simulink model "SecRwRtStZeroTrgtPosSelc"  (R2018b)
settings: Solver=FixedStepDiscrete  StartTime=0.0  StopTime=10.0  RelTol=1e-3
undefined symbols (not defined in the file or in its folder): KeSMSw6SAcsEntrySecRwRtStCushnFrtUpwdDnwdPos_Val, KeSMSw6SAcsEntrySecRwRtStCushnFrtUpwdDnwdPosMax_Val, KeSMSw6SAcsEntrySecRwRtStCushnFrtUpwdDnwdPosMin_Val, KeSMSw6SRecoveryMdSecRwRtStCushnFrtUpwdDnwdPos_Val, KeSMSw6SRecoveryMdSecRwRtStCushnFrtUpwdDnwdPosMax_Val, KeSMSw6SRecoveryMdSecRwRtStCushnFrtUpwdDnwdPosMin_Val, KeSMSwAcsEntrySecRwRtStCushnFrtIUpwdDnwdPos_Val, KeSMSwAcsEntrySecRwRtStCushnFrtIUpwdDnwdPosMax_Val, KeSMSwAcsEntrySecRwRtStCushnFrtIUpwdDnwdPosMin_Val, KeSMSwAcsMd8SecRwRtStCushnFrtUpwdDnwdPos_Val, KeSMSwAcsMd8SecRwRtStCushnFrtUpwdDnwdPosMax_Val, KeSMSwAcsMd8SecRwRtStCushnFrtUpwdDnwdPosMin_Val, KeSMSwAcsMd9SecRwRtStCushnFrtUpwdDnwdPos_Val, KeSMSwAcsMd9SecRwRtStCushnFrtUpwdDnwdPosMax_Val, KeSMSwAcsMd9SecRwRtStCushnFrtUpwdDnwdPosMin_Val, KeSMSwRecoveryMdSecRwRtStCushnFrtInwdOtwdPos_Val, KeSMSwRecoveryMdSecRwRtStCushnFrtInwdOtwdPosMax_Val, KeSMSwRecoveryMdSecRwRtStCushnFrtInwdOtwdPosMin_Val, KeSMSwRecoveryMdSecRwRtStCushnFrtUpwdDnwdPos_Val, KeSMSwRecoveryMdSecRwRtStCushnFrtUpwdDnwdPosMax_Val, KeSMSwRecoveryMdSecRwRtStCushnFrtUpwdDnwdPosMin_Val, KeSMSwSecRwRtStZeroEnTrig5576sBitMask_Val, KeSMSwSecRwRtStZeroEnTrig557BitMask_Val
libraries: TrgtPosSelcLib x4
settings Model: Creator=sn2xws  LastModifiedBy=sn2xws
settings Model: ModifiedHistory=|
  | 2024.7.8 V3.0.0 557模式流程V1.9
  | 2024.8.14 V3.0.1增加6s版本bitmask标定
settings DataIOCC: SaveFormat=StructureWithTime
settings OptimizationCC: DefaultParameterBehavior=Inlined  EnhancedBackFolding=on  PassReuseOutputArgsAs=Individual arguments  ZeroExternalMemoryAtStartup=off  ZeroInternalMemoryAtStartup=off  OptimizeBlockOrder=speed  DifferentSizesBufferReuse=on  OptimizationCustomize=off
settings DebuggingCC: ParameterTunabilityLossMsg=error
settings SFSimCC: MATLABDynamicMemAlloc=off
settings RTWCC: SystemTargetFile=autosar.tlc  GenCodeOnly=on  TemplateMakefile=ert_default_tmf  Description=AUTOSAR  GenerateReport=on  IncludeHyperlinkInReport=on  LaunchReport=on  GenerateTraceInfo=on  GenerateTraceReport=on  GenerateTraceReportSl=on  GenerateTraceReportSf=on  GenerateTraceReportEml=on
settings CodeAppCC: ForceParamTrailComments=on  IgnoreCustomStorageClasses=off  OperatorAnnotations=on  SimulinkDataObjDesc=on  SFDataObjDesc=on  InsertBlockDesc=on
settings STFCustomTargetCC: TargetLangStandard=C99 (ISO)  MultiwordLength=256  ParMdlRefBuildCompliant=on  CompOptLevelCompliant=on  IncludeMdlTerminateFcn=off  CombineOutputUpdateFcns=on  SuppressErrorStatus=on  ERTCustomFileBanners=on  SupportNonFinite=off  SupportComplex=off  SupportContinuousTime=off  SupportNonInlinedSFcns=off  RemoveResetFunc=on  MATLABClassNameForMDSCustomization=Simulink.SoftwareTarget.ERTCustomization  AutosarCompliant=on  UseToolchainInfoCompliant=on  LookupTableObjectStructAxisOrder=2,1,3,4,...  LUTObjectStructOrderEvenSpacing=Size,Table,Breakpoints  SystemTargetFile=autosar.tlc
settings ERTTargetCC: TargetLangStandard=C99 (ISO)  ConcurrentExecutionCompliant=off  IncludeMdlTerminateFcn=off  SuppressErrorStatus=on  SupportNonFinite=off  SupportComplex=off  ModelStepFunctionPrototypeControlCompliant=off  CPPClassGenCompliant=off  AutosarCompliant=on  LookupTableObjectStructAxisOrder=2,1,3,4,...  LUTObjectStructOrderEvenSpacing=Size,Table,Breakpoints  InlinedParameterPlacement=NonHierarchical  ERTCustomFileTemplate=example_file_process.tlc  ERTFilePackagingFormat=Compact

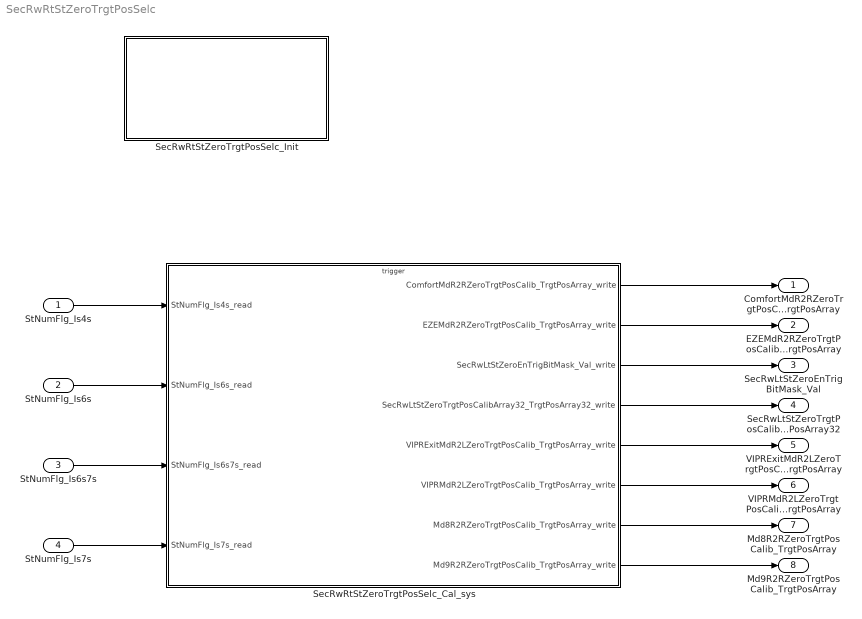
== system SecRwRtStZeroTrgtPosSelc ==
  StNumFlg_Is4s : Inport  OutDataTypeStr=boolean  PortDimensions=1
  StNumFlg_Is6s : Inport  Port=2  OutDataTypeStr=boolean  PortDimensions=1
  StNumFlg_Is6s7s : Inport  Port=3  OutDataTypeStr=boolean  PortDimensions=1
  StNumFlg_Is7s : Inport  Port=4  OutDataTypeStr=boolean  PortDimensions=1
  SecRwRtStZeroTrgtPosSelc_Cal_sys : Subsystem
  SecRwRtStZeroTrgtPosSelc_Init : Subsystem
  ComfortMdR2RZeroTrgtPosCalib_TrgtPosArray : Outport  Description=|  OutDataTypeStr=uint16  PortDimensions=3
      | 0:Pos
      | 1:Max
      | 2:Min
  EZEMdR2RZeroTrgtPosCalib_TrgtPosArray : Outport  Description=|  Port=2  OutDataTypeStr=uint16  PortDimensions=3
      | 0:Pos
      | 1:Max
      | 2:Min
  SecRwLtStZeroEnTrigBitMask_Val : Outport  Port=3  OutDataTypeStr=uint32  PortDimensions=1
  SecRwLtStZeroTrgtPosCalibArray32_TrgtPosArray32 : Outport  Description=|  Port=4  OutDataTypeStr=uint16  PortDimensions=96
      | 0:Pos
      | 1:Max
      | 2:Min
  VIPRExitMdR2LZeroTrgtPosCalib_TrgtPosArray : Outport  Description=|  Port=5  OutDataTypeStr=uint16  PortDimensions=3
      | 0:Pos
      | 1:Max
      | 2:Min
  VIPRMdR2LZeroTrgtPosCalib_TrgtPosArray : Outport  Description=|  Port=6  OutDataTypeStr=uint16  PortDimensions=3
      | 0:Pos
      | 1:Max
      | 2:Min
  Md8R2RZeroTrgtPosCalib_TrgtPosArray : Outport  Description=|  Port=7  OutDataTypeStr=uint16  PortDimensions=3
      | 0:Pos
      | 1:Max
      | 2:Min
  Md9R2RZeroTrgtPosCalib_TrgtPosArray : Outport  Description=|  Port=8  OutDataTypeStr=uint16  PortDimensions=3
      | 0:Pos
      | 1:Max
      | 2:Min
  wires:
  StNumFlg_Is4s/1 -> SecRwRtStZeroTrgtPosSelc_Cal_sys/1(StNumFlg_Is4s_read)
  StNumFlg_Is6s/1 -> SecRwRtStZeroTrgtPosSelc_Cal_sys/2(StNumFlg_Is6s_read)
  StNumFlg_Is6s7s/1 -> SecRwRtStZeroTrgtPosSelc_Cal_sys/3(StNumFlg_Is6s7s_read)
  StNumFlg_Is7s/1 -> SecRwRtStZeroTrgtPosSelc_Cal_sys/4(StNumFlg_Is7s_read)
  SecRwRtStZeroTrgtPosSelc_Cal_sys/1(ComfortMdR2RZeroTrgtPosCalib_TrgtPosArray_write) -> ComfortMdR2RZeroTrgtPosCalib_TrgtPosArray/1
  SecRwRtStZeroTrgtPosSelc_Cal_sys/2(EZEMdR2RZeroTrgtPosCalib_TrgtPosArray_write) -> EZEMdR2RZeroTrgtPosCalib_TrgtPosArray/1
  SecRwRtStZeroTrgtPosSelc_Cal_sys/3(SecRwLtStZeroEnTrigBitMask_Val_write) -> SecRwLtStZeroEnTrigBitMask_Val/1
  SecRwRtStZeroTrgtPosSelc_Cal_sys/4(SecRwLtStZeroTrgtPosCalibArray32_TrgtPosArray32_write) -> SecRwLtStZeroTrgtPosCalibArray32_TrgtPosArray32/1
  SecRwRtStZeroTrgtPosSelc_Cal_sys/5(VIPRExitMdR2LZeroTrgtPosCalib_TrgtPosArray_write) -> VIPRExitMdR2LZeroTrgtPosCalib_TrgtPosArray/1
  SecRwRtStZeroTrgtPosSelc_Cal_sys/6(VIPRMdR2LZeroTrgtPosCalib_TrgtPosArray_write) -> VIPRMdR2LZeroTrgtPosCalib_TrgtPosArray/1
  SecRwRtStZeroTrgtPosSelc_Cal_sys/7(Md8R2RZeroTrgtPosCalib_TrgtPosArray_write) -> Md8R2RZeroTrgtPosCalib_TrgtPosArray/1
  SecRwRtStZeroTrgtPosSelc_Cal_sys/8(Md9R2RZeroTrgtPosCalib_TrgtPosArray_write) -> Md9R2RZeroTrgtPosCalib_TrgtPosArray/1

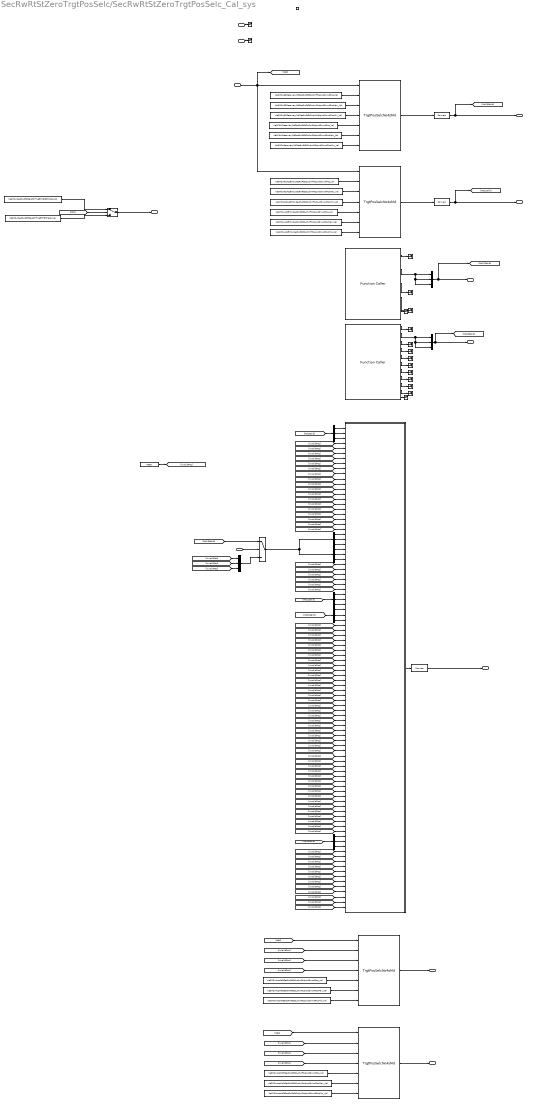
== system SecRwRtStZeroTrgtPosSelc/SecRwRtStZeroTrgtPosSelc_Cal_sys ==
  StNumFlg_Is4s_read : Inport
  StNumFlg_Is6s_read : Inport  Port=2
  StNumFlg_Is6s7s_read : Inport  Port=3
  StNumFlg_Is7s_read : Inport  Port=4
  function : TriggerPort  TriggerType=function-call  IsSimulinkFunction=on  FunctionName=SecRwRtStZeroTrgtPosSelc_Cal  VariantControl=(inherit)
  Constant : Constant  Value=4095  OutDataTypeStr=uint16
  Data Type Conversion : DataTypeConversion
  Data Type Conversion1 : DataTypeConversion
  Data Type Conversion3 : DataTypeConversion
  Demux{,1..5} (6 alike) : Demux  Outputs=3
  Mux : Mux  Inputs=3
  Mux1 : Mux  Inputs=3
  Mux2 : Mux  Inputs=3
  PA_KeSMSw6SAcsEntrySecRwRtStCushnFrtUpwdDnwdPosMax_Val : Constant  Value=KeSMSw6SAcsEntrySecRwRtStCushnFrtUpwdDnwdPosMax_Val
  PA_KeSMSw6SAcsEntrySecRwRtStCushnFrtUpwdDnwdPosMin_Val : Constant  Value=KeSMSw6SAcsEntrySecRwRtStCushnFrtUpwdDnwdPosMin_Val
  PA_KeSMSw6SAcsEntrySecRwRtStCushnFrtUpwdDnwdPos_Val : Constant  Value=KeSMSw6SAcsEntrySecRwRtStCushnFrtUpwdDnwdPos_Val
  PA_KeSMSw6SRecoveryMdSecRwRtStCushnFrtUpwdDnwdPosMax_Val : Constant  Value=KeSMSw6SRecoveryMdSecRwRtStCushnFrtUpwdDnwdPosMax_Val
  PA_KeSMSw6SRecoveryMdSecRwRtStCushnFrtUpwdDnwdPosMin_Val : Constant  Value=KeSMSw6SRecoveryMdSecRwRtStCushnFrtUpwdDnwdPosMin_Val
  PA_KeSMSw6SRecoveryMdSecRwRtStCushnFrtUpwdDnwdPos_Val : Constant  Value=KeSMSw6SRecoveryMdSecRwRtStCushnFrtUpwdDnwdPos_Val
  PA_KeSMSwAcsEntrySecRwRtStCushnFrtIUpwdDnwdPosMax_Val : Constant  Value=KeSMSwAcsEntrySecRwRtStCushnFrtIUpwdDnwdPosMax_Val
  PA_KeSMSwAcsEntrySecRwRtStCushnFrtIUpwdDnwdPosMin_Val : Constant  Value=KeSMSwAcsEntrySecRwRtStCushnFrtIUpwdDnwdPosMin_Val
  PA_KeSMSwAcsEntrySecRwRtStCushnFrtIUpwdDnwdPos_Val : Constant  Value=KeSMSwAcsEntrySecRwRtStCushnFrtIUpwdDnwdPos_Val
  PA_KeSMSwAcsMd8SecRwRtStCushnFrtUpwdDnwdPosMax_Val : Constant  Value=KeSMSwAcsMd8SecRwRtStCushnFrtUpwdDnwdPosMax_Val
  PA_KeSMSwAcsMd8SecRwRtStCushnFrtUpwdDnwdPosMin_Val : Constant  Value=KeSMSwAcsMd8SecRwRtStCushnFrtUpwdDnwdPosMin_Val
  PA_KeSMSwAcsMd8SecRwRtStCushnFrtUpwdDnwdPos_Val : Constant  Value=KeSMSwAcsMd8SecRwRtStCushnFrtUpwdDnwdPos_Val
  PA_KeSMSwAcsMd9SecRwRtStCushnFrtUpwdDnwdPosMax_Val : Constant  Value=KeSMSwAcsMd9SecRwRtStCushnFrtUpwdDnwdPosMax_Val
  PA_KeSMSwAcsMd9SecRwRtStCushnFrtUpwdDnwdPosMin_Val : Constant  Value=KeSMSwAcsMd9SecRwRtStCushnFrtUpwdDnwdPosMin_Val
  PA_KeSMSwAcsMd9SecRwRtStCushnFrtUpwdDnwdPos_Val : Constant  Value=KeSMSwAcsMd9SecRwRtStCushnFrtUpwdDnwdPos_Val
  PA_KeSMSwRecoveryMdSecRwRtStCushnFrtUpwdDnwdPosMax_Val : Constant  Value=KeSMSwRecoveryMdSecRwRtStCushnFrtUpwdDnwdPosMax_Val
  PA_KeSMSwRecoveryMdSecRwRtStCushnFrtUpwdDnwdPosMin_Val : Constant  Value=KeSMSwRecoveryMdSecRwRtStCushnFrtUpwdDnwdPosMin_Val
  PA_KeSMSwRecoveryMdSecRwRtStCushnFrtUpwdDnwdPos_Val : Constant  Value=KeSMSwRecoveryMdSecRwRtStCushnFrtUpwdDnwdPos_Val
  PA_KeSMSwSecRwRtStZeroEnTrig5576sBitMask_Val : Constant  Value=KeSMSwSecRwRtStZeroEnTrig5576sBitMask_Val
  PA_KeSMSwSecRwRtStZeroEnTrig557BitMask_Val : Constant  Value=KeSMSwSecRwRtStZeroEnTrig557BitMask_Val
  Subsystem : Subsystem
  Switch : Switch  Criteria=u2 > Threshold
  Switch1 : Switch  Criteria=u2 > Threshold
  Terminator{,1..11} (12 alike) : Terminator
  Terminator_{1,3,21..22} (4 alike) : Terminator
  TrgtPosSelcNot4sMotor{,1..3} (4 alike) : TrgtPosSelcLib/TrgtPosSelcNo4sMd  SystemSampleTime=-1
  VIPR557TrgtPos_Get : FunctionCaller  FunctionPrototype=[SecRwLtStBkReclnTrgtPos,SecRwLtStZeroTrgtPos,SecRwLtStLgrstUpwdDnwdTrgtPos,SecRwLtStLgrstInwdOtwdTrgtPos,SecRwLtStFwdBkwdTrgtPos] = VIPR557TrgtPos_Get()  OutputArgumentSpecifications=uint16(1), uint16(1), uint16(1), uint16(1), uint16(1)
  VIPRExit557TrgtPos_Get : FunctionCaller  FunctionPrototype=[SecRwRtStBkReclnTrgtPos,SecRwRtStZeroTrgtPos,SecRwRtStLgrstUpwdDnwdTrgtPos,SecRwRtStLgrstInwdOtwdTrgtPos,ThdRwLtStBkReclnTrgtPos,ThdRwLtStFwdBkwdTrgtPos,ThdRwRtStBkReclnTrgtPos,ThdRwRtStFwdBkwdTrgtPos,PassStBkReclnTrgtPos,PassStFwdBkwdTrgtPos,SecRwRtStFwdBkwdTrgtPos] = VIPRExit557TrgtPos_Get()  OutputArgumentSpecifications=uint16(1), uint16(1), uint16(1), uint16(1), uint16(1), uint16(1), uint16(1), uint16(1), uint16(1), uint16(1), uint16(1)
  ComfortMdR2RZeroTrgtPosCalib_TrgtPosArray_write : Outport
      settings: EnsureOutportIsVirtual=on
  EZEMdR2RZeroTrgtPosCalib_TrgtPosArray_write : Outport  Port=2
      settings: EnsureOutportIsVirtual=on
  SecRwLtStZeroEnTrigBitMask_Val_write : Outport  Port=3
      settings: EnsureOutportIsVirtual=on
  SecRwLtStZeroTrgtPosCalibArray32_TrgtPosArray32_write : Outport  Port=4
      settings: EnsureOutportIsVirtual=on
  VIPRExitMdR2LZeroTrgtPosCalib_TrgtPosArray_write : Outport  Port=5
      settings: EnsureOutportIsVirtual=on
  VIPRMdR2LZeroTrgtPosCalib_TrgtPosArray_write : Outport  Port=6
      settings: EnsureOutportIsVirtual=on
  Md8R2RZeroTrgtPosCalib_TrgtPosArray_write : Outport  Port=7
      settings: EnsureOutportIsVirtual=on
  Md9R2RZeroTrgtPosCalib_TrgtPosArray_write : Outport  Port=8
      settings: EnsureOutportIsVirtual=on
  wires:
  StNumFlg_Is4s_read/1 -> Terminator_1/1
  StNumFlg_Is6s7s_read/1 -> Terminator_3/1
  Data Type Conversion/1 -> [Md13Calib], ComfortMdR2RZeroTrgtPosCalib_TrgtPosArray_write/1
  TrgtPosSelcNot4sMotor/1 -> Data Type Conversion/1
  Data Type Conversion1/1 -> [Md1Calib], EZEMdR2RZeroTrgtPosCalib_TrgtPosArray_write/1
  TrgtPosSelcNot4sMotor1/1 -> Data Type Conversion1/1
  PA_KeSMSw6SRecoveryMdSecRwRtStCushnFrtUpwdDnwdPos_Val/1 -> TrgtPosSelcNot4sMotor/2
  PA_KeSMSw6SRecoveryMdSecRwRtStCushnFrtUpwdDnwdPosMax_Val/1 -> TrgtPosSelcNot4sMotor/3
  PA_KeSMSw6SRecoveryMdSecRwRtStCushnFrtUpwdDnwdPosMin_Val/1 -> TrgtPosSelcNot4sMotor/4
  PA_KeSMSwRecoveryMdSecRwRtStCushnFrtUpwdDnwdPos_Val/1 -> TrgtPosSelcNot4sMotor/5
  PA_KeSMSwRecoveryMdSecRwRtStCushnFrtUpwdDnwdPosMax_Val/1 -> TrgtPosSelcNot4sMotor/6
  PA_KeSMSwRecoveryMdSecRwRtStCushnFrtUpwdDnwdPosMin_Val/1 -> TrgtPosSelcNot4sMotor/7
  PA_KeSMSw6SAcsEntrySecRwRtStCushnFrtUpwdDnwdPos_Val/1 -> TrgtPosSelcNot4sMotor1/2
  PA_KeSMSw6SAcsEntrySecRwRtStCushnFrtUpwdDnwdPosMax_Val/1 -> TrgtPosSelcNot4sMotor1/3
  PA_KeSMSw6SAcsEntrySecRwRtStCushnFrtUpwdDnwdPosMin_Val/1 -> TrgtPosSelcNot4sMotor1/4
  PA_KeSMSwAcsEntrySecRwRtStCushnFrtIUpwdDnwdPos_Val/1 -> TrgtPosSelcNot4sMotor1/5
  PA_KeSMSwAcsEntrySecRwRtStCushnFrtIUpwdDnwdPosMax_Val/1 -> TrgtPosSelcNot4sMotor1/6
  PA_KeSMSwAcsEntrySecRwRtStCushnFrtIUpwdDnwdPosMin_Val/1 -> TrgtPosSelcNot4sMotor1/7
  Mux/1 -> [Md12Calib], VIPRMdR2LZeroTrgtPosCalib_TrgtPosArray_write/1
  [invalidPos] -> Subsystem/62(Md21PosMax)
  [invalidPos] -> Subsystem/45(Md15PosMin)
  Demux1/2 -> Subsystem/83(Md28PosMax)
  [invalidPos] -> Subsystem/74(Md25PosMax)
  [invalidPos] -> Subsystem/88(Md30Pos)
  [invalidPos] -> Subsystem/68(Md23PosMax)
  [invalidPos] -> Subsystem/57(Md19PosMin)
  [invalidPos] -> Subsystem/44(Md15PosMax)
  [Md28Calib] -> Demux1/1
  [invalidPos] -> Subsystem/7(Md3Pos)
  [invalidPos] -> Subsystem/15(Md5PosMin)
  Demux1/3 -> Subsystem/84(Md28PosMin)
  [invalidPos] -> Subsystem/94(Md32Pos)
  Demux1/1 -> Subsystem/82(Md28Pos)
  [invalidPos] -> Subsystem/56(Md19PosMax)
  Demux3/3 -> Subsystem/39(Md13PosMin)
  [invalidPos] -> Subsystem/14(Md5PosMax)
  [invalidPos] -> Subsystem/49(Md17Pos)
  [invalidPos] -> Subsystem/80(Md27PosMax)
  [invalidPos] -> Subsystem/47(Md16PosMax)
  [Md12Calib] -> Demux/1
  [invalidPos] -> Subsystem/75(Md25PosMin)
  [invalidPos] -> Subsystem/77(Md26PosMax)
  [invalidPos] -> Subsystem/87(Md29PosMin)
  [invalidPos] -> Subsystem/86(Md29PosMax)
  [invalidPos] -> Subsystem/50(Md17PosMax)
  Subsystem/1(CalibArray32) -> Data Type Conversion3/1
  [invalidPos] -> Subsystem/79(Md27Pos)
  [invalidPos] -> Subsystem/59(Md20PosMax)
  [invalidPos] -> Subsystem/76(Md26Pos)
  [invalidPos] -> Subsystem/78(Md26PosMin)
  [invalidPos] -> Subsystem/66(Md22PosMin)
  [invalidPos] -> Subsystem/72(Md24PosMin)
  Demux3/2 -> Subsystem/38(Md13PosMax)
  [invalidPos] -> Subsystem/71(Md24PosMax)
  [invalidPos] -> Subsystem/17(Md6PosMax)
  [invalidPos] -> Subsystem/95(Md32PosMax)
  [invalidPos] -> Subsystem/53(Md18PosMax)
  [invalidPos] -> Subsystem/64(Md22Pos)
  [invalidPos] -> Subsystem/10(Md4Pos)
  [invalidPos] -> Subsystem/61(Md21Pos)
  [invalidPos] -> Subsystem/55(Md19Pos)
  [invalidPos] -> Subsystem/85(Md29Pos)
  [invalidPos] -> Subsystem/19(Md7Pos)
  [invalidPos] -> Subsystem/96(Md32PosMin)
  [invalidPos] -> Subsystem/67(Md23Pos)
  [invalidPos] -> Subsystem/29(Md10PosMax)
  Data Type Conversion3/1 -> SecRwLtStZeroTrgtPosCalibArray32_TrgtPosArray32_write/1
  [invalidPos] -> Subsystem/30(Md10PosMin)
  [invalidPos] -> Subsystem/16(Md6Pos)
  [invalidPos] -> Subsystem/28(Md10Pos)
  [invalidPos] -> Subsystem/12(Md4PosMin)
  [invalidPos] -> Subsystem/21(Md7PosMin)
  [invalidPos] -> Subsystem/6(Md2PosMin)
  [invalidPos] -> Subsystem/69(Md23PosMin)
  [invalidPos] -> Subsystem/4(Md2Pos)
  [invalidPos] -> Subsystem/81(Md27PosMin)
  [invalidPos] -> Subsystem/11(Md4PosMax)
  [invalidPos] -> Subsystem/73(Md25Pos)
  [invalidPos] -> Subsystem/5(Md2PosMax)
  [invalidPos] -> Subsystem/51(Md17PosMin)
  [invalidPos] -> Subsystem/65(Md22PosMax)
  [invalidPos] -> Subsystem/48(Md16PosMin)
  [invalidPos] -> Subsystem/70(Md24Pos)
  [invalidPos] -> Subsystem/52(Md18Pos)
  Demux/3 -> Subsystem/36(Md12PosMin)
  [invalidPos] -> Subsystem/9(Md3PosMin)
  [invalidPos] -> Subsystem/63(Md21PosMin)
  [invalidPos] -> Subsystem/33(Md11PosMin)
  [invalidPos] -> Subsystem/31(Md11Pos)
  [invalidPos] -> Subsystem/46(Md16Pos)
  Demux3/1 -> Subsystem/37(Md13Pos)
  [invalidPos] -> Subsystem/8(Md3PosMax)
  [invalidPos] -> Subsystem/13(Md5Pos)
  Demux/1 -> Subsystem/34(Md12Pos)
  Demux/2 -> Subsystem/35(Md12PosMax)
  Constant/1 -> [invalidPos]
  [invalidPos] -> Subsystem/54(Md18PosMin)
  [invalidPos] -> Subsystem/18(Md6PosMin)
  [invalidPos] -> Subsystem/42(Md14PosMin)
  [invalidPos] -> Subsystem/40(Md14Pos)
  Demux2/3 -> Subsystem/3(Md1Min)
  [invalidPos] -> Subsystem/43(Md15Pos)
  Demux2/1 -> Subsystem/1(Md1Pos)
  [invalidPos] -> Subsystem/60(Md20PosMin)
  [invalidPos] -> Subsystem/58(Md20Pos)
  [invalidPos] -> Subsystem/41(Md14PosMax)
  Demux2/2 -> Subsystem/2(Md1Max)
  [invalidPos] -> Subsystem/20(Md7PosMax)
  [invalidPos] -> Subsystem/32(Md11PosMax)
  [invalidPos] -> Subsystem/91(Md31Pos)
  [invalidPos] -> Subsystem/92(Md31PosMax)
  [invalidPos] -> Subsystem/93(Md31PosMin)
  [invalidPos] -> Subsystem/90(Md30PosMin)
  [invalidPos] -> Subsystem/89(Md30PosMax)
  VIPR557TrgtPos_Get/2 -> Mux/3, Mux/2, Mux/1
  VIPRExit557TrgtPos_Get/2 -> Mux1/1, Mux1/2, Mux1/3
  Mux1/1 -> [Md28Calib], VIPRExitMdR2LZeroTrgtPosCalib_TrgtPosArray_write/1
  VIPRExit557TrgtPos_Get/4 -> Terminator/1
  VIPRExit557TrgtPos_Get/1 -> Terminator2/1
  VIPRExit557TrgtPos_Get/3 -> Terminator1/1
  VIPRExit557TrgtPos_Get/5 -> Terminator3/1
  VIPRExit557TrgtPos_Get/6 -> Terminator4/1
  VIPRExit557TrgtPos_Get/7 -> Terminator5/1
  VIPRExit557TrgtPos_Get/8 -> Terminator6/1
  VIPRExit557TrgtPos_Get/9 -> Terminator7/1
  VIPRExit557TrgtPos_Get/10 -> Terminator8/1
  VIPR557TrgtPos_Get/1 -> Terminator9/1
  VIPR557TrgtPos_Get/3 -> Terminator10/1
  VIPR557TrgtPos_Get/4 -> Terminator11/1
  [Md1Calib] -> Demux2/1
  [Md13Calib] -> Demux3/1
  Demux4/1 -> Subsystem/22(Md8Pos)
  Demux4/2 -> Subsystem/23(Md8PosMax)
  Demux4/3 -> Subsystem/24(Md8PosMin)
  Demux5/3 -> Subsystem/27(Md9PosMin)
  Demux5/2 -> Subsystem/26(Md9PosMax)
  Demux5/1 -> Subsystem/25(Md9Pos)
  StNumFlg_Is7s_read/1 -> Switch/2
  [Md13Calib] -> Switch/1
  [invalidPos] -> Mux2/1
  [invalidPos] -> Mux2/2
  [invalidPos] -> Mux2/3
  Mux2/1 -> Switch/3
  Switch/1 -> Demux5/1, Demux4/1
  PA_KeSMSwAcsMd9SecRwRtStCushnFrtUpwdDnwdPosMax_Val/1 -> TrgtPosSelcNot4sMotor3/6
  PA_KeSMSwAcsMd9SecRwRtStCushnFrtUpwdDnwdPosMin_Val/1 -> TrgtPosSelcNot4sMotor3/7
  PA_KeSMSwAcsMd9SecRwRtStCushnFrtUpwdDnwdPos_Val/1 -> TrgtPosSelcNot4sMotor3/5
  VIPR557TrgtPos_Get/5 -> Terminator_21/1
  VIPRExit557TrgtPos_Get/11 -> Terminator_22/1
  TrgtPosSelcNot4sMotor3/1 -> Md9R2RZeroTrgtPosCalib_TrgtPosArray_write/1
  TrgtPosSelcNot4sMotor2/1 -> Md8R2RZeroTrgtPosCalib_TrgtPosArray_write/1
  StNumFlg_Is6s_read/1 -> [Is6s], TrgtPosSelcNot4sMotor1/1, TrgtPosSelcNot4sMotor/1
  [Is6s] -> TrgtPosSelcNot4sMotor2/1
  [invalidPos] -> TrgtPosSelcNot4sMotor2/2
  [invalidPos] -> TrgtPosSelcNot4sMotor2/3
  [invalidPos] -> TrgtPosSelcNot4sMotor2/4
  PA_KeSMSwAcsMd8SecRwRtStCushnFrtUpwdDnwdPos_Val/1 -> TrgtPosSelcNot4sMotor2/5
  PA_KeSMSwAcsMd8SecRwRtStCushnFrtUpwdDnwdPosMax_Val/1 -> TrgtPosSelcNot4sMotor2/6
  PA_KeSMSwAcsMd8SecRwRtStCushnFrtUpwdDnwdPosMin_Val/1 -> TrgtPosSelcNot4sMotor2/7
  [Is6s] -> TrgtPosSelcNot4sMotor3/1
  [invalidPos] -> TrgtPosSelcNot4sMotor3/2
  [invalidPos] -> TrgtPosSelcNot4sMotor3/3
  [invalidPos] -> TrgtPosSelcNot4sMotor3/4
  PA_KeSMSwSecRwRtStZeroEnTrig5576sBitMask_Val/1 -> Switch1/1
  Switch1/1 -> SecRwLtStZeroEnTrigBitMask_Val_write/1
  [Is6s] -> Switch1/2
  PA_KeSMSwSecRwRtStZeroEnTrig557BitMask_Val/1 -> Switch1/3

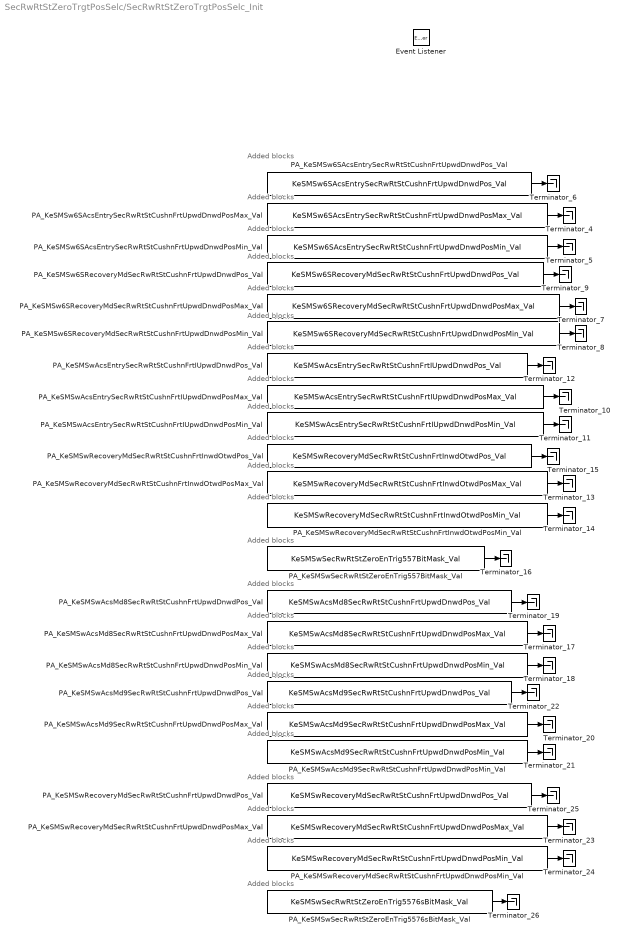
== system SecRwRtStZeroTrgtPosSelc/SecRwRtStZeroTrgtPosSelc_Init ==
  note: Added blocks
  note: Added blocks
  note: Added blocks
  note: Added blocks
  note: Added blocks
  note: Added blocks
  note: Added blocks
  note: Added blocks
  note: Added blocks
  note: Added blocks
  note: Added blocks
  note: Added blocks
  note: Added blocks
  note: Added blocks
  note: Added blocks
  note: Added blocks
  note: Added blocks
  note: Added blocks
  note: Added blocks
  note: Added blocks
  note: Added blocks
  note: Added blocks
  note: Added blocks
  Event Listener : EventListener  EventName=reset
  PA_KeSMSw6SAcsEntrySecRwRtStCushnFrtUpwdDnwdPosMax_Val : Constant  Value=KeSMSw6SAcsEntrySecRwRtStCushnFrtUpwdDnwdPosMax_Val
  PA_KeSMSw6SAcsEntrySecRwRtStCushnFrtUpwdDnwdPosMin_Val : Constant  Value=KeSMSw6SAcsEntrySecRwRtStCushnFrtUpwdDnwdPosMin_Val
  PA_KeSMSw6SAcsEntrySecRwRtStCushnFrtUpwdDnwdPos_Val : Constant  Value=KeSMSw6SAcsEntrySecRwRtStCushnFrtUpwdDnwdPos_Val
  PA_KeSMSw6SRecoveryMdSecRwRtStCushnFrtUpwdDnwdPosMax_Val : Constant  Value=KeSMSw6SRecoveryMdSecRwRtStCushnFrtUpwdDnwdPosMax_Val
  PA_KeSMSw6SRecoveryMdSecRwRtStCushnFrtUpwdDnwdPosMin_Val : Constant  Value=KeSMSw6SRecoveryMdSecRwRtStCushnFrtUpwdDnwdPosMin_Val
  PA_KeSMSw6SRecoveryMdSecRwRtStCushnFrtUpwdDnwdPos_Val : Constant  Value=KeSMSw6SRecoveryMdSecRwRtStCushnFrtUpwdDnwdPos_Val
  PA_KeSMSwAcsEntrySecRwRtStCushnFrtIUpwdDnwdPosMax_Val : Constant  Value=KeSMSwAcsEntrySecRwRtStCushnFrtIUpwdDnwdPosMax_Val
  PA_KeSMSwAcsEntrySecRwRtStCushnFrtIUpwdDnwdPosMin_Val : Constant  Value=KeSMSwAcsEntrySecRwRtStCushnFrtIUpwdDnwdPosMin_Val
  PA_KeSMSwAcsEntrySecRwRtStCushnFrtIUpwdDnwdPos_Val : Constant  Value=KeSMSwAcsEntrySecRwRtStCushnFrtIUpwdDnwdPos_Val
  PA_KeSMSwAcsMd8SecRwRtStCushnFrtUpwdDnwdPosMax_Val : Constant  Value=KeSMSwAcsMd8SecRwRtStCushnFrtUpwdDnwdPosMax_Val
  PA_KeSMSwAcsMd8SecRwRtStCushnFrtUpwdDnwdPosMin_Val : Constant  Value=KeSMSwAcsMd8SecRwRtStCushnFrtUpwdDnwdPosMin_Val
  PA_KeSMSwAcsMd8SecRwRtStCushnFrtUpwdDnwdPos_Val : Constant  Value=KeSMSwAcsMd8SecRwRtStCushnFrtUpwdDnwdPos_Val
  PA_KeSMSwAcsMd9SecRwRtStCushnFrtUpwdDnwdPosMax_Val : Constant  Value=KeSMSwAcsMd9SecRwRtStCushnFrtUpwdDnwdPosMax_Val
  PA_KeSMSwAcsMd9SecRwRtStCushnFrtUpwdDnwdPosMin_Val : Constant  Value=KeSMSwAcsMd9SecRwRtStCushnFrtUpwdDnwdPosMin_Val
  PA_KeSMSwAcsMd9SecRwRtStCushnFrtUpwdDnwdPos_Val : Constant  Value=KeSMSwAcsMd9SecRwRtStCushnFrtUpwdDnwdPos_Val
  PA_KeSMSwRecoveryMdSecRwRtStCushnFrtInwdOtwdPosMax_Val : Constant  Value=KeSMSwRecoveryMdSecRwRtStCushnFrtInwdOtwdPosMax_Val
  PA_KeSMSwRecoveryMdSecRwRtStCushnFrtInwdOtwdPosMin_Val : Constant  Value=KeSMSwRecoveryMdSecRwRtStCushnFrtInwdOtwdPosMin_Val
  PA_KeSMSwRecoveryMdSecRwRtStCushnFrtInwdOtwdPos_Val : Constant  Value=KeSMSwRecoveryMdSecRwRtStCushnFrtInwdOtwdPos_Val
  PA_KeSMSwRecoveryMdSecRwRtStCushnFrtUpwdDnwdPosMax_Val : Constant  Value=KeSMSwRecoveryMdSecRwRtStCushnFrtUpwdDnwdPosMax_Val
  PA_KeSMSwRecoveryMdSecRwRtStCushnFrtUpwdDnwdPosMin_Val : Constant  Value=KeSMSwRecoveryMdSecRwRtStCushnFrtUpwdDnwdPosMin_Val
  PA_KeSMSwRecoveryMdSecRwRtStCushnFrtUpwdDnwdPos_Val : Constant  Value=KeSMSwRecoveryMdSecRwRtStCushnFrtUpwdDnwdPos_Val
  PA_KeSMSwSecRwRtStZeroEnTrig5576sBitMask_Val : Constant  Value=KeSMSwSecRwRtStZeroEnTrig5576sBitMask_Val
  PA_KeSMSwSecRwRtStZeroEnTrig557BitMask_Val : Constant  Value=KeSMSwSecRwRtStZeroEnTrig557BitMask_Val
  Terminator_{4..26} (23 alike) : Terminator
  wires:
  PA_KeSMSw6SAcsEntrySecRwRtStCushnFrtUpwdDnwdPosMax_Val/1 -> Terminator_4/1
  PA_KeSMSw6SAcsEntrySecRwRtStCushnFrtUpwdDnwdPosMin_Val/1 -> Terminator_5/1
  PA_KeSMSw6SAcsEntrySecRwRtStCushnFrtUpwdDnwdPos_Val/1 -> Terminator_6/1
  PA_KeSMSw6SRecoveryMdSecRwRtStCushnFrtUpwdDnwdPosMax_Val/1 -> Terminator_7/1
  PA_KeSMSw6SRecoveryMdSecRwRtStCushnFrtUpwdDnwdPosMin_Val/1 -> Terminator_8/1
  PA_KeSMSw6SRecoveryMdSecRwRtStCushnFrtUpwdDnwdPos_Val/1 -> Terminator_9/1
  PA_KeSMSwAcsEntrySecRwRtStCushnFrtIUpwdDnwdPosMax_Val/1 -> Terminator_10/1
  PA_KeSMSwAcsEntrySecRwRtStCushnFrtIUpwdDnwdPosMin_Val/1 -> Terminator_11/1
  PA_KeSMSwAcsEntrySecRwRtStCushnFrtIUpwdDnwdPos_Val/1 -> Terminator_12/1
  PA_KeSMSwRecoveryMdSecRwRtStCushnFrtInwdOtwdPosMax_Val/1 -> Terminator_13/1
  PA_KeSMSwRecoveryMdSecRwRtStCushnFrtInwdOtwdPosMin_Val/1 -> Terminator_14/1
  PA_KeSMSwRecoveryMdSecRwRtStCushnFrtInwdOtwdPos_Val/1 -> Terminator_15/1
  PA_KeSMSwSecRwRtStZeroEnTrig557BitMask_Val/1 -> Terminator_16/1
  PA_KeSMSwAcsMd8SecRwRtStCushnFrtUpwdDnwdPosMax_Val/1 -> Terminator_17/1
  PA_KeSMSwAcsMd8SecRwRtStCushnFrtUpwdDnwdPosMin_Val/1 -> Terminator_18/1
  PA_KeSMSwAcsMd8SecRwRtStCushnFrtUpwdDnwdPos_Val/1 -> Terminator_19/1
  PA_KeSMSwAcsMd9SecRwRtStCushnFrtUpwdDnwdPosMax_Val/1 -> Terminator_20/1
  PA_KeSMSwAcsMd9SecRwRtStCushnFrtUpwdDnwdPosMin_Val/1 -> Terminator_21/1
  PA_KeSMSwAcsMd9SecRwRtStCushnFrtUpwdDnwdPos_Val/1 -> Terminator_22/1
  PA_KeSMSwRecoveryMdSecRwRtStCushnFrtUpwdDnwdPosMax_Val/1 -> Terminator_23/1
  PA_KeSMSwRecoveryMdSecRwRtStCushnFrtUpwdDnwdPosMin_Val/1 -> Terminator_24/1
  PA_KeSMSwRecoveryMdSecRwRtStCushnFrtUpwdDnwdPos_Val/1 -> Terminator_25/1
  PA_KeSMSwSecRwRtStZeroEnTrig5576sBitMask_Val/1 -> Terminator_26/1

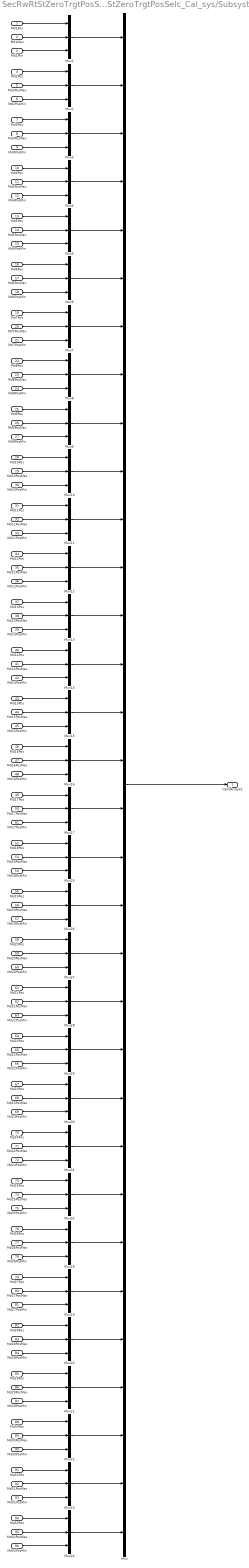
== system SecRwRtStZeroTrgtPosSelc/SecRwRtStZeroTrgtPosSelc_Cal_sys/Subsystem ==
  Md1Pos : Inport
  Md1Max : Inport  Port=2
  Md1Min : Inport  Port=3
  Md2Pos : Inport  Port=4
  Md2PosMax : Inport  Port=5
  Md2PosMin : Inport  Port=6
  Md3Pos : Inport  Port=7
  Md3PosMax : Inport  Port=8
  Md3PosMin : Inport  Port=9
  Md4Pos : Inport  Port=10
  Md4PosMax : Inport  Port=11
  Md4PosMin : Inport  Port=12
  Md5Pos : Inport  Port=13
  Md5PosMax : Inport  Port=14
  Md5PosMin : Inport  Port=15
  Md6Pos : Inport  Port=16
  Md6PosMax : Inport  Port=17
  Md6PosMin : Inport  Port=18
  Md7Pos : Inport  Port=19
  Md7PosMax : Inport  Port=20
  Md7PosMin : Inport  Port=21
  Md8Pos : Inport  Port=22
  Md8PosMax : Inport  Port=23
  Md8PosMin : Inport  Port=24
  Md9Pos : Inport  Port=25
  Md9PosMax : Inport  Port=26
  Md9PosMin : Inport  Port=27
  Md10Pos : Inport  Port=28
  Md10PosMax : Inport  Port=29
  Md10PosMin : Inport  Port=30
  Md11Pos : Inport  Port=31
  Md11PosMax : Inport  Port=32
  Md11PosMin : Inport  Port=33
  Md12Pos : Inport  Port=34
  Md12PosMax : Inport  Port=35
  Md12PosMin : Inport  Port=36
  Md13Pos : Inport  Port=37
  Md13PosMax : Inport  Port=38
  Md13PosMin : Inport  Port=39
  Md14Pos : Inport  Port=40
  Md14PosMax : Inport  Port=41
  Md14PosMin : Inport  Port=42
  Md15Pos : Inport  Port=43
  Md15PosMax : Inport  Port=44
  Md15PosMin : Inport  Port=45
  Md16Pos : Inport  Port=46
  Md16PosMax : Inport  Port=47
  Md16PosMin : Inport  Port=48
  Md17Pos : Inport  Port=49
  Md17PosMax : Inport  Port=50
  Md17PosMin : Inport  Port=51
  Md18Pos : Inport  Port=52
  Md18PosMax : Inport  Port=53
  Md18PosMin : Inport  Port=54
  Md19Pos : Inport  Port=55
  Md19PosMax : Inport  Port=56
  Md19PosMin : Inport  Port=57
  Md20Pos : Inport  Port=58
  Md20PosMax : Inport  Port=59
  Md20PosMin : Inport  Port=60
  Md21Pos : Inport  Port=61
  Md21PosMax : Inport  Port=62
  Md21PosMin : Inport  Port=63
  Md22Pos : Inport  Port=64
  Md22PosMax : Inport  Port=65
  Md22PosMin : Inport  Port=66
  Md23Pos : Inport  Port=67
  Md23PosMax : Inport  Port=68
  Md23PosMin : Inport  Port=69
  Md24Pos : Inport  Port=70
  Md24PosMax : Inport  Port=71
  Md24PosMin : Inport  Port=72
  Md25Pos : Inport  Port=73
  Md25PosMax : Inport  Port=74
  Md25PosMin : Inport  Port=75
  Md26Pos : Inport  Port=76
  Md26PosMax : Inport  Port=77
  Md26PosMin : Inport  Port=78
  Md27Pos : Inport  Port=79
  Md27PosMax : Inport  Port=80
  Md27PosMin : Inport  Port=81
  Md28Pos : Inport  Port=82
  Md28PosMax : Inport  Port=83
  Md28PosMin : Inport  Port=84
  Md29Pos : Inport  Port=85
  Md29PosMax : Inport  Port=86
  Md29PosMin : Inport  Port=87
  Md30Pos : Inport  Port=88
  Md30PosMax : Inport  Port=89
  Md30PosMin : Inport  Port=90
  Md31Pos : Inport  Port=91
  Md31PosMax : Inport  Port=92
  Md31PosMin : Inport  Port=93
  Md32Pos : Inport  Port=94
  Md32PosMax : Inport  Port=95
  Md32PosMin : Inport  Port=96
  Mux : Mux  Inputs=32
  Mux{1..32} (32 alike) : Mux  Inputs=3
  CalibArray32 : Outport
  wires:
  Md22PosMax/1 -> Mux29/2
  Md3PosMin/1 -> Mux3/3
  Mux13/1 -> Mux/13
  Md13Pos/1 -> Mux13/1
  Mux30/1 -> Mux/23
  Md2PosMax/1 -> Mux2/2
  Md12PosMin/1 -> Mux12/3
  Md15PosMax/1 -> Mux15/2
  Md17Pos/1 -> Mux17/1
  Mux20/1 -> Mux/28
  Mux27/1 -> Mux/20
  Mux11/1 -> Mux/11
  Mux31/1 -> Mux/24
  Mux24/1 -> Mux/32
  Md8PosMin/1 -> Mux8/3
  Mux7/1 -> Mux/7
  Md20Pos/1 -> Mux27/1
  Mux6/1 -> Mux/6
  Md2PosMin/1 -> Mux2/3
  Md2Pos/1 -> Mux2/1
  Md5Pos/1 -> Mux5/1
  Md4PosMax/1 -> Mux4/2
  Mux25/1 -> Mux/18
  Md5PosMin/1 -> Mux5/3
  Md16PosMin/1 -> Mux16/3
  Md12PosMax/1 -> Mux12/2
  Mux32/1 -> Mux/25
  Md15PosMin/1 -> Mux15/3
  Mux15/1 -> Mux/15
  Mux16/1 -> Mux/16
  Mux21/1 -> Mux/29
  Md27PosMax/1 -> Mux19/2
  Md28Pos/1 -> Mux20/1
  Md13PosMin/1 -> Mux13/3
  Mux29/1 -> Mux/22
  Md8Pos/1 -> Mux8/1
  Mux23/1 -> Mux/31
  Mux22/1 -> Mux/30
  Mux12/1 -> Mux/12
  Md24Pos/1 -> Mux31/1
  Mux9/1 -> Mux/9
  Mux8/1 -> Mux/8
  Md9Pos/1 -> Mux9/1
  Mux3/1 -> Mux/3
  Md6PosMin/1 -> Mux6/3
  Mux17/1 -> Mux/17
  Md6Pos/1 -> Mux6/1
  Mux14/1 -> Mux/14
  Mux1/1 -> Mux/1
  Md10Pos/1 -> Mux10/1
  Md9PosMax/1 -> Mux9/2
  Mux26/1 -> Mux/19
  Mux18/1 -> Mux/26
  Mux28/1 -> Mux/21
  Mux2/1 -> Mux/2
  Mux19/1 -> Mux/27
  Mux10/1 -> Mux/10
  Mux5/1 -> Mux/5
  Md23PosMin/1 -> Mux30/3
  Md4PosMin/1 -> Mux4/3
  Md7PosMin/1 -> Mux7/3
  Md4Pos/1 -> Mux4/1
  Mux4/1 -> Mux/4
  Md13PosMax/1 -> Mux13/2
  Md6PosMax/1 -> Mux6/2
  Md5PosMax/1 -> Mux5/2
  Md14PosMax/1 -> Mux14/2
  Md14PosMin/1 -> Mux14/3
  Md23PosMax/1 -> Mux30/2
  Md1Min/1 -> Mux1/3
  Md8PosMax/1 -> Mux8/2
  Md23Pos/1 -> Mux30/1
  Md1Pos/1 -> Mux1/1
  Md1Max/1 -> Mux1/2
  Md9PosMin/1 -> Mux9/3
  Md7PosMax/1 -> Mux7/2
  Md20PosMin/1 -> Mux27/3
  Md7Pos/1 -> Mux7/1
  Md10PosMax/1 -> Mux10/2
  Md10PosMin/1 -> Mux10/3
  Md15Pos/1 -> Mux15/1
  Md30PosMax/1 -> Mux22/2
  Md11PosMax/1 -> Mux11/2
  Md12Pos/1 -> Mux12/1
  Md11PosMin/1 -> Mux11/3
  Md11Pos/1 -> Mux11/1
  Md14Pos/1 -> Mux14/1
  Md16Pos/1 -> Mux16/1
  Md24PosMin/1 -> Mux31/3
  Md16PosMax/1 -> Mux16/2
  Md32PosMin/1 -> Mux24/3
  Md27Pos/1 -> Mux19/1
  Md32PosMax/1 -> Mux24/2
  Md18Pos/1 -> Mux25/1
  Md19Pos/1 -> Mux26/1
  Md19PosMax/1 -> Mux26/2
  Md21Pos/1 -> Mux28/1
  Md27PosMin/1 -> Mux19/3
  Md26PosMax/1 -> Mux18/2
  Md26PosMin/1 -> Mux18/3
  Md31Pos/1 -> Mux23/1
  Md25Pos/1 -> Mux32/1
  Md28PosMin/1 -> Mux20/3
  Md25PosMin/1 -> Mux32/3
  Md25PosMax/1 -> Mux32/2
  Md17PosMin/1 -> Mux17/3
  Md32Pos/1 -> Mux24/1
  Md24PosMax/1 -> Mux31/2
  Md18PosMax/1 -> Mux25/2
  Md21PosMin/1 -> Mux28/3
  Md30PosMin/1 -> Mux22/3
  Md21PosMax/1 -> Mux28/2
  Md22Pos/1 -> Mux29/1
  Md18PosMin/1 -> Mux25/3
  Md26Pos/1 -> Mux18/1
  Md20PosMax/1 -> Mux27/2
  Md31PosMin/1 -> Mux23/3
  Md29Pos/1 -> Mux21/1
  Md19PosMin/1 -> Mux26/3
  Md29PosMin/1 -> Mux21/3
  Md30Pos/1 -> Mux22/1
  Md17PosMax/1 -> Mux17/2
  Md28PosMax/1 -> Mux20/2
  Md22PosMin/1 -> Mux29/3
  Md31PosMax/1 -> Mux23/2
  Md29PosMax/1 -> Mux21/2
  Mux/1 -> CalibArray32/1
  Md3Pos/1 -> Mux3/1
  Md3PosMax/1 -> Mux3/2
